simulink model "stm32f4_basicpwm_demo"  (Simulink 10.3)
settings: Solver=FixedStepDiscrete  StartTime=0.0  StopTime=10.0  RelTol=1e-3
PreLoadFcn:
  | waijung.modelPreload; % Required for working with Waijung Blockset. Do not remove.
undefined symbols (not defined in the file or in its folder): HSEOSC, Link, LQFP64, ST, STM32F446RE
libraries: stm32f4_io_lib x1, stm32f4_device_config_lib x1
CloseFcn:
  | waijung.modelClose; % Required for working with Waijung Blockset. Do not remove.
settings Model: Creator=Krisada  LastModifiedBy=dudekpob
settings Model: SuppressorTable=|
  | <?xml version="1.0" encoding="UTF-8" standalone="yes" ?>
  | <!DOCTYPE boost_serialization>
  | <boost_serialization signature="serialization::archive" version="17">
  | <DiagnosticSuppressor class_id="0" tracking_level="0" version="7">
  | 	<Table class_id="1" tracking_level="0" version="0">
  | 		<count>1</count>
  | 		<bucket_count>8</bucket_count>
  | 		<item_version>0</item_version>
  | 		<item class_id="2" tracking_level="0" version="0">
  | 			<first class_id="3" tracking_level="0" version="7">
  | 				<Source class_id="4" tracking_level="0" version="0">
  | 					<count>1</count>
  | 					<item_version>0</item_version>
  | 					<item>5</item>
  | 				</Source>
  | 			</first>
  | 			<second class_id="5" tracking_level="0" version="7">
  | 				<SuppressedData class_id="6" tracking_level="0" version="0">
  | 					<count>2</count>
  | 					<bucket_count>8</bucket_count>
  | 					<item_version>0</item_version>
  | 					<item class_id="7" tracking_level="0" version="0">
  | 						<first class_id="8" tracking_level="0" version="7">
  | 							<ID>SimulinkFixedPoint:util:Overflowoccurred</ID>
  | 							<Cause>
  | 								<Source>
  | 									<count>0</count>
  | 									<item_version>0</item_version>
  | 								</Source>
  | 							</Cause>
  | 						</first>
  | 						<second class_id="9" tracking_level="0" version="7">
  | 							<Comment></Comment>
  | 							<User></User>
  | 							<LastModified class_id="10" tracking_level="0" version="0">
  | 								<ptime_date class_id="11" tracking_level="0" version="0">
  | 									<date>20160608</date>
  | 								</ptime_date>
  | 								<ptime_time_duration class_id="12" tracking_level="0" version="1">
  | 									<is_special>0</is_special>
  | 									<time_duration_hours>15</time_duration_hours>
  | 									<time_duration_minutes>23</time_duration_minutes>
  | 									<time_duration_seconds>17</time_duration_seconds>
  | 									<time_duration_fractional_seconds>0</time_duration_fractional_seconds>
  | 								</ptime_time_duration>
  | 							</LastModified>
  | 							<SuppressionType>1</SuppressionType>
  | 						</second>
  | 					</item>
  | 					<item>
  | 						<first>
  | 							<ID>Simulink:DataType:WarningOverFlowDetected</ID>
  | 							<Cause>
  | 								<Source>
  | 									<count>0</count>
  | 									<item_version>0</item_version>
  | 								</Source>
  | 							</Cause>
  | 						</first>
  | 						<second>
  | 							<Comment></Comment>
  | 							<User></User>
  | 							<LastModified>
  | 								<ptime_date>
  | 									<date>20160608</date>
  | 								</ptime_date>
  | 								<ptime_time_duration>
  | 									<is_special>0</is_special>
  | 									<time_duration_hours>15</time_duration_hours>
  | 									<time_duration_minutes>23</time_duration_minutes>
  | 									<time_duration_seconds>17</time_duration_seconds>
  | 									<time_duration_fractional_seconds>0</time_duration_fractional_seconds>
  | 								</ptime_time_duration>
  | 							</LastModified>
  | 							<SuppressionType>1</SuppressionType>
  | 						</second>
  | 					</item>
  | 				</SuppressedData>
  | 			</second>
  | 		</item>
  | 	</Table>
  | </DiagnosticSuppressor>
  | 
  | </boost_serialization>
  | 
  | </boost_serialization>
settings DataIOCC: LimitDataPoints=on
settings OptimizationCC: LifeSpan=1  EfficientTunableParamExpr=on
settings DebuggingCC: SolverPrmCheckMsg=warning
settings HardwareCC: ProdEndianess=LittleEndian  ProdHWDeviceType=ARM Compatible->Cortex - M4  TargetEndianess=LittleEndian  TargetHWDeviceType=ARM Compatible->Cortex - M4
settings SFSimCC: MATLABDynamicMemAlloc=off
settings RTWCC: Description=STM32F4 Target  SystemTargetFile=stm32f4.tlc  GenerateMakefile=off  TemplateMakefile=ert_default_tmf  RetainRTWFile=on
settings CodeAppCC: IgnoreCustomStorageClasses=off  CustomSymbolStrType=$N$R$M  InternalIdentifier=Classic
settings STFCustomTargetCC: ModelReferenceCompliant=off  CombineOutputUpdateFcns=on  ERTCustomFileBanners=on  SupportContinuousTime=off  SupportNonInlinedSFcns=off  RemoveResetFunc=on  MATLABClassNameForMDSCustomization=Simulink.SoftwareTarget.ERTCustomization  GRTInterface=off  SystemTargetFile=stm32f4.tlc
settings ERTTargetCC: MultiwordLength=2048  ModelReferenceCompliant=off  ParMdlRefBuildCompliant=off  CompOptLevelCompliant=off  ConcurrentExecutionCompliant=off  ModelStepFunctionPrototypeControlCompliant=off  CPPClassGenCompliant=off  UseToolchainInfoCompliant=off  ExtModeMexFile=noextcomm  ERTSrcFileBannerTemplate=stm32f4_code_template.cgt  ERTHdrFileBannerTemplate=stm32f4_code_template.cgt  ERTDataSrcFileTemplate=stm32f4_code_template.cgt  ERTDataHdrFileTemplate=stm32f4_code_template.cgt  ERTCustomFileTemplate=stm32f4_file_process.tlc  ConvertIfToSwitch=off  SuppressUnreachableDefaultCases=off

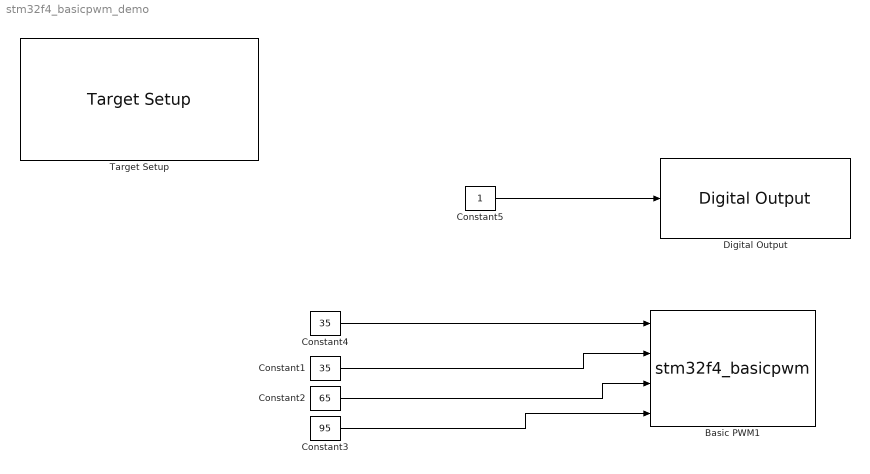
== system stm32f4_basicpwm_demo ==
  Basic PWM1 : S-Function  FunctionName=stm32f4_basicpwm  Parameters=timer,pwmperiod,ch1pin,ch2pin,ch3pin,ch4pin,sampletime,sampletimestr,blockid,apb,portstr,pinstr,pinmat,timarr,timprescale,chmat,polaritystr  SFunctionDeploymentMode=off  EnableBusSupport=off  mask(stm32f4_basicpwm){timer=2, pwmperiod=0.02, polarity=Active High, polaritystr=TIM_OCPolarity_High, ch1pin=A0, ch2pin=A1, ch3pin=A2, ch4pin=A3, sampletime=0.1, sampletimestr=-1, blockid=BasicPWM1, portpinstr=A0,A1,A2,A3, enablecustomportlabel=off, cinputportlabel=In1, In2, In3, In4, coutputportlabel=0, apb=1, portstr=["A"], pinstr=["GPIO_Pin_0 | GPIO_Pin_1 | GPIO_Pin_2 | GPIO_Pin_3"], pinmat=[4 0 1 2 3], timarr=64284, timprescale=27, chmat=[1  2  3  4]}
      mask prompts: pwmperiod "PWM Period (seconds)"; ch1pin "Channel 1"; ch2pin "Channel 2"; ch3pin "Channel 3"; ch4pin "Channel 4"; sampletime "Sample time (sec)"; sampletimestr "Compiled sample time (sec) in string"; portpinstr "Port pin string"; enablecustomportlabel "Enable custom port labels"; cinputportlabel "Custom input port labels (Ex. In1, In2, In3)"; coutputportlabel "Custom output port labels (Ex. Out1, Out2, Out3)"; portstr "Port string"; pinstr "Pin string"; pinmat "Pin matrix"; timarr "Timer ARR"; timprescale "Timer PRESCALE"; chmat "Channel order"
      mask help:
      | This block implements basic Edge-aligned Pulse Width Modulation (PWM) generation.
      | All timers are 16-bit. The PWM period is fixed (per timer).
      mask init:
      | stm32f4_basicpwm_callback('init');
      mask Help: web(fullfile(waijungdocroot,'stm32f4_basicpwm.htm'),'-browser')
      mask TypeOptions timer: 1 | 2 | 3 | 4 | 5 | 8 | 9 | 10 | 11 | 12 | 13 | 14
      mask Callback timer: stm32f4_basicpwm_callback('timer');
      mask Callback pwmperiod: stm32f4_basicpwm_callback('pwmperiod');
      mask TypeOptions polarity: Active High | Active Low
      mask Callback polarity: stm32f4_basicpwm_callback('polarity');
      mask TypeOptions ch1pin: Not available - Do not use | A0 | A5 | A15
      mask Callback ch1pin: stm32f4_basicpwm_callback('ch1pin');
      mask TypeOptions ch2pin: Not available - Do not use | A1 | B3
      mask Callback ch2pin: stm32f4_basicpwm_callback('ch2pin');
      mask TypeOptions ch3pin: Not available - Do not use | A2 | B10
      mask Callback ch3pin: stm32f4_basicpwm_callback('ch3pin');
      mask TypeOptions ch4pin: Not available - Do not use | A3 | B11
      mask Callback ch4pin: stm32f4_basicpwm_callback('ch4pin');
      mask Callback sampletime: stm32f4_basicpwm_callback('sampletime');
      mask Callback sampletimestr: stm32f4_basicpwm_callback('sampletimestr');
      mask Callback blockid: stm32f4_basicpwm_callback('blockid');
      mask Callback enablecustomportlabel: stm32f4_basicpwm_callback('enablecustomportlabel');
      mask Display: text(0.95, 0.5, 'Timer: 2\nPolarity: Active High\nPeriod (sec) 0.02\nTs (sec): -1','ver','middle','hor','right');port_label('input', 1,'CH1 (A0)');port_label('input', 2,'CH2 (A1)');port_label('input', 3,'CH3 (A2)');port_label('input', 4,'CH4 (A3)')
  Constant1 : Constant  Value=35
  Constant2 : Constant  Value=65
  Constant3 : Constant  Value=95
  Constant4 : Constant  Value=35
  Constant5 : Constant  OutDataTypeStr=boolean
  Digital Output : stm32f4_io_lib/Digital Output  use_bitband=on  port=A  speed=100  porttype=Push Pull  porttypestr=PP  use_pin0=off  use_pin1=off  use_pin2=off  use_pin3=off  use_pin4=off  use_pin5=on  use_pin6=off  use_pin7=off  use_pin8=off  use_pin9=off  use_pin10=off  use_pin11=off  use_pin12=off  use_pin13=off  use_pin14=off  use_pin15=off  pinstr=GPIO_Pin_5  usedpinarray="[0  0  0  0  0  1  0  0  0  0  0  0  0  0  0  0]"  bitbandingstr="#define DigitalOutput_A5 Peripheral_BB(GPIOA->ODR, 5)  /* Output pin */"  sampletime=-1  sampletimestr=-1  blockid=DigitalOutput  enablecustomportlabel=off  globalinit=off  cinputportlabel=In1, In2  coutputportlabel=0
      settings: SourceProductName=Waijung Blockset
  Target Setup : stm32f4_device_config_lib/Target Setup  Priority=100  compiler=GNU ARM  previous_compiler=GNU ARM  mcu=STM32F446RE (LQFP64)  mcustr=STM32F446RE  clockconfig=HSEOSC-8MHz  system_stm32f4xx_c_path=C:\STM32_matlab\waijung_18.11a\targets\stm32f4_target\stm32f4\utils\system_stm32f4xx_default\STM32F446xx\hseosc8mhz  showmemoryconfiguration=off  stacksize=0x400  heapsize=0x200  enableautocompiledownload=on  fullchiperase=on  programmerinterface=ST-Link  editctrlstr=on  compilercontrolstr=$(patsubst %, -I%, .) -mcpu=cortex-m4 -mthumb -mthumb-interwork -mfloat-abi=hard -mfpu=fpv4-sp-d16 -ffast-math -Wall -Wextra -Ofast  assemblercontrolstr=$(patsubst %, -I%, .) -mcpu=cortex-m4 -mthumb -mthumb-interwork -mfloat-abi=hard -mfpu=fpv4-sp-d16 -ffast-math -Wall -Wextra -Ofast -Wa,-amhls=$(<:.s=.lst) -D__STACK_SIZE=$(STACK_SIZE) -D__HEAP_SIZE=$(HEAP_SIZE)  linkercontrolstr=-T$(LD_SCRIPT) -g -Wl,-Map=$(MAP),--cref,--no-warn-mismatch -mcpu=cortex-m4 -mthumb -mthumb-interwork -mfloat-abi=hard -mfpu=fpv4-sp-d16  runafterdownload=on  execprofile=None  profileruart=3  profilerbaud=115200  profilertxpin=D8  profilerinitstr=0.01,180000000,1800000,115200,0  manualsetsampletime=off  sampletime=0.01  blockid=TargetSetup  systickreloadvalue=1800000  hseval=8000000  lastprofileruart=3  hclk=180000000  flashorigin=0x8000000  flashlength=512k  ramorigin=0x20000000  ramlength=128k  useextram=off
      settings: SourceProductName=Waijung Blockset
  wires:
  Constant4/1 -> Basic PWM1/1
  Constant1/1 -> Basic PWM1/2
  Constant2/1 -> Basic PWM1/3
  Constant3/1 -> Basic PWM1/4
  Constant5/1 -> Digital Output/1
